simulink model "AirplanePorts"  (Simulink 7.9)
settings: Solver=ode3  StartTime=0.0  StopTime=10.0  FixedStep=0.01  RelTol=1e-3
libraries: orocos_taskcontext x3
settings Model: Creator=meyer  LastModifiedBy=meyer

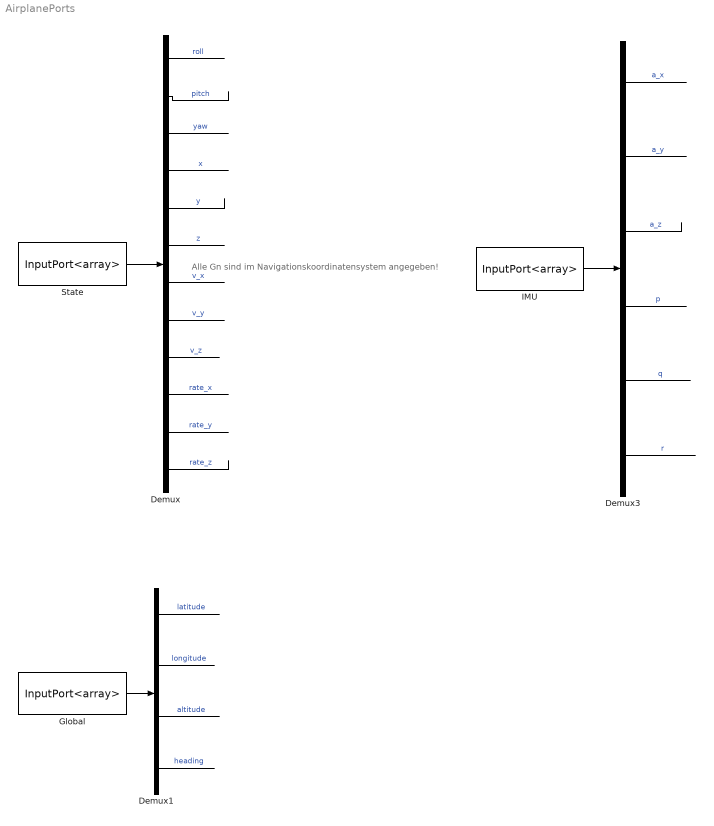
== system AirplanePorts ==
  note: Alle Gn sind im
      | Navigationskoordinatensystem angegeben!
  Demux : Demux  Outputs=12
  Demux1 : Demux
  Demux3 : Demux  Outputs=6
  Global : orocos_taskcontext/InputPort<array>  dpdesc=Port's Description  dpvalue=zeros(1,4)
      settings: AttributesFormatString=Value=%<dpvalue>
  IMU : orocos_taskcontext/InputPort<array>  dpdesc=Port's Description  dpvalue=zeros(1,6)
      settings: AttributesFormatString=Value=%<dpvalue>
  State : orocos_taskcontext/InputPort<array>  dpdesc=Port's Description  dpvalue=zeros(1,12)
      settings: AttributesFormatString=Value=%<dpvalue>
  wires:
  State/1 -> Demux/1
  IMU/1 -> Demux3/1
  Demux/1 -> ?  "roll"
  Demux/2 -> ?  "pitch"
  Demux/3 -> ?  "yaw"
  Demux/4 -> ?  "x"
  Demux/5 -> ?  "y"
  Demux/6 -> ?  "z"
  Demux/7 -> ?  "v_x"
  Demux/8 -> ?  "v_y"
  Demux/9 -> ?  "v_z"
  Demux/10 -> ?  "rate_x"
  Demux/11 -> ?  "rate_y"
  Demux/12 -> ?  "rate_z"
  Demux3/1 -> ?  "a_x"
  Demux3/2 -> ?  "a_y"
  Demux3/3 -> ?  "a_z"
  Demux3/4 -> ?  "p"
  Demux3/5 -> ?  "q"
  Demux3/6 -> ?  "r"
  Global/1 -> Demux1/1
  Demux1/1 -> ?  "latitude"
  Demux1/2 -> ?  "longitude"
  Demux1/3 -> ?  "altitude"
  Demux1/4 -> ?  "heading"
